simulink model "test_mdl_NI"  (R2018a)
settings: Solver=VariableStepAuto  StartTime=0.0  StopTime=10.0  RelTol=1e-3
(part 16 of 24)

== system test_mdl_NI/CAN_Signal/ABS_ESC/TrailerBrakeData_0x412/VehPtch_An_Dsply ==
  in : Inport
  out : Outport
  wires:
  in/1 -> out/1

== system test_mdl_NI/CAN_Signal/ABS_ESC/TrailerBrakeData_0x412/VehRol_An_Dsply ==
  in : Inport
  out : Outport
  wires:
  in/1 -> out/1

== system test_mdl_NI/CAN_Signal/ABS_ESC/WheelData_0x216/BrkObdData_No_Actl ==
  in : Inport
  out : Outport
  wires:
  in/1 -> out/1

== system test_mdl_NI/CAN_Signal/ABS_ESC/WheelData_0x216/BrkObdIndex_No_Actl ==
  in : Inport
  out : Outport
  wires:
  in/1 -> out/1

== system test_mdl_NI/CAN_Signal/ABS_ESC/WheelData_0x216/WhlDirFl_D_Actl ==
  in : Inport
  out : Outport
  wires:
  in/1 -> out/1

== system test_mdl_NI/CAN_Signal/ABS_ESC/WheelData_0x216/WhlDirFr_D_Actl ==
  in : Inport
  out : Outport
  wires:
  in/1 -> out/1

== system test_mdl_NI/CAN_Signal/ABS_ESC/WheelData_0x216/WhlDirRl_D_Actl ==
  in : Inport
  out : Outport
  wires:
  in/1 -> out/1

== system test_mdl_NI/CAN_Signal/ABS_ESC/WheelData_0x216/WhlDirRr_D_Actl ==
  in : Inport
  out : Outport
  wires:
  in/1 -> out/1

== system test_mdl_NI/CAN_Signal/ABS_ESC/WheelData_0x216/WhlRotatFl_No_Cnt ==
  in : Inport
  out : Outport
  wires:
  in/1 -> out/1

== system test_mdl_NI/CAN_Signal/ABS_ESC/WheelData_0x216/WhlRotatFr_No_Cnt ==
  in : Inport
  out : Outport
  wires:
  in/1 -> out/1

== system test_mdl_NI/CAN_Signal/ABS_ESC/WheelData_0x216/WhlRotatRl_No_Cnt ==
  in : Inport
  out : Outport
  wires:
  in/1 -> out/1

== system test_mdl_NI/CAN_Signal/ABS_ESC/WheelData_0x216/WhlRotatRr_No_Cnt ==
  in : Inport
  out : Outport
  wires:
  in/1 -> out/1

== system test_mdl_NI/CAN_Signal/ABS_ESC/WheelSpeed_0x217/WhlFl_W_Meas ==
  in : Inport
  out : Outport
  wires:
  in/1 -> out/1

== system test_mdl_NI/CAN_Signal/ABS_ESC/WheelSpeed_0x217/WhlFr_W_Meas ==
  in : Inport
  out : Outport
  wires:
  in/1 -> out/1

== system test_mdl_NI/CAN_Signal/ABS_ESC/WheelSpeed_0x217/WhlRl_W_Meas ==
  in : Inport
  out : Outport
  wires:
  in/1 -> out/1

== system test_mdl_NI/CAN_Signal/ABS_ESC/WheelSpeed_0x217/WhlRr_W_Meas ==
  in : Inport
  out : Outport
  wires:
  in/1 -> out/1

== system test_mdl_NI/CAN_Signal/ADAS/ACCDATA/AccBrkDecel_B_Rq ==
  in : Inport
  out : Outport
  wires:
  in/1 -> out/1

== system test_mdl_NI/CAN_Signal/ADAS/ACCDATA/AccBrkPrchg_B_Rq ==
  in : Inport
  out : Outport
  wires:
  in/1 -> out/1

== system test_mdl_NI/CAN_Signal/ADAS/ACCDATA/AccBrkTot_A_Rq ==
  in : Inport
  out : Outport
  wires:
  in/1 -> out/1

== system test_mdl_NI/CAN_Signal/ADAS/ACCDATA/AccCancl_B_Rq ==
  in : Inport
  out : Outport
  wires:
  in/1 -> out/1

== system test_mdl_NI/CAN_Signal/ADAS/ACCDATA/AccPrpl_A_Rq ==
  in : Inport
  out : Outport
  wires:
  in/1 -> out/1

== system test_mdl_NI/CAN_Signal/ADAS/ACCDATA/AccPrpl_A_Rq1 ==
  in : Inport
  out : Outport
  wires:
  in/1 -> out/1

== system test_mdl_NI/CAN_Signal/ADAS/ACCDATA/AccStopStat_B_Rq ==
  in : Inport
  out : Outport
  wires:
  in/1 -> out/1

== system test_mdl_NI/CAN_Signal/ADAS/ACCDATA/CmbbEngTqMn_B_Rq ==
  in : Inport
  out : Outport
  wires:
  in/1 -> out/1

== system test_mdl_NI/CAN_Signal/ADAS/ACCDATA_2/CmbbBaSens_D_Rq ==
  in : Inport
  out : Outport
  wires:
  in/1 -> out/1

== system test_mdl_NI/CAN_Signal/ADAS/ACCDATA_2/CmbbBrkDecel_A_Rq ==
  in : Inport
  out : Outport
  wires:
  in/1 -> out/1

== system test_mdl_NI/CAN_Signal/ADAS/ACCDATA_2/CmbbBrkDecel_B_Rq ==
  in : Inport
  out : Outport
  wires:
  in/1 -> out/1

== system test_mdl_NI/CAN_Signal/ADAS/ACCDATA_2/CmbbBrkPrchg_D_Rq ==
  in : Inport
  out : Outport
  wires:
  in/1 -> out/1

== system test_mdl_NI/CAN_Signal/BCM/BCM_Lamp_Stat_0x3C3/BrkWarnInd_B_Rq ==
  in : Inport
  out : Outport
  wires:
  in/1 -> out/1

== system test_mdl_NI/CAN_Signal/BCM/BCM_Lamp_Stat_0x3C3/Brk_Fluid_Lvl_Low ==
  in : Inport
  out : Outport
  wires:
  in/1 -> out/1

== system test_mdl_NI/CAN_Signal/BCM/BCM_Lamp_Stat_0x3C3/Courtesy_BSave_Stat ==
  in : Inport
  out : Outport
  wires:
  in/1 -> out/1

== system test_mdl_NI/CAN_Signal/BCM/BCM_Lamp_Stat_0x3C3/Courtesy_Delay_Status ==
  in : Inport
  out : Outport
  wires:
  in/1 -> out/1

== system test_mdl_NI/CAN_Signal/BCM/BCM_Lamp_Stat_0x3C3/CrnrLghtLeft_Pc_Rq ==
  in : Inport
  out : Outport
  wires:
  in/1 -> out/1

== system test_mdl_NI/CAN_Signal/BCM/BCM_Lamp_Stat_0x3C3/CrnrLghtRight_Pc_Rq ==
  in : Inport
  out : Outport
  wires:
  in/1 -> out/1

== system test_mdl_NI/CAN_Signal/BCM/BCM_Lamp_Stat_0x3C3/DayRnngLampOn_B_Stat ==
  in : Inport
  out : Outport
  wires:
  in/1 -> out/1

== system test_mdl_NI/CAN_Signal/BCM/BCM_Lamp_Stat_0x3C3/DrTgateLck_D_Stat ==
  in : Inport
  out : Outport
  wires:
  in/1 -> out/1

== system test_mdl_NI/CAN_Signal/BCM/BCM_Lamp_Stat_0x3C3/Dr_Courtesy_Light_Stat ==
  in : Inport
  out : Outport
  wires:
  in/1 -> out/1

== system test_mdl_NI/CAN_Signal/BCM/BCM_Lamp_Stat_0x3C3/HeadLampLoActv_B_Stat ==
  in : Inport
  out : Outport
  wires:
  in/1 -> out/1

== system test_mdl_NI/CAN_Signal/BCM/BCM_Lamp_Stat_0x3C3/HeadLampLoFlOn_B_Stat ==
  in : Inport
  out : Outport
  wires:
  in/1 -> out/1

== system test_mdl_NI/CAN_Signal/BCM/BCM_Lamp_Stat_0x3C3/HeadLampLoFrOn_B_Stat ==
  in : Inport
  out : Outport
  wires:
  in/1 -> out/1

== system test_mdl_NI/CAN_Signal/BCM/BCM_Lamp_Stat_0x3C3/HeadLampLoOut_B_Stat ==
  in : Inport
  out : Outport
  wires:
  in/1 -> out/1

== system test_mdl_NI/CAN_Signal/BCM/BCM_Lamp_Stat_0x3C3/HeadLghtHiFdbck_D_Stat ==
  in : Inport
  out : Outport
  wires:
  in/1 -> out/1

== system test_mdl_NI/CAN_Signal/BCM/BCM_Lamp_Stat_0x3C3/HeadLghtHiOn_B_Stat ==
  in : Inport
  out : Outport
  wires:
  in/1 -> out/1

== system test_mdl_NI/CAN_Signal/BCM/BCM_Lamp_Stat_0x3C3/HeadLghtSwtch_D_Stat ==
  in : Inport
  out : Outport
  wires:
  in/1 -> out/1

== system test_mdl_NI/CAN_Signal/BCM/BCM_Lamp_Stat_0x3C3/Headlamp_On_Wrning_Cmd ==
  in : Inport
  out : Outport
  wires:
  in/1 -> out/1

== system test_mdl_NI/CAN_Signal/BCM/BCM_Lamp_Stat_0x3C3/HomeSafeLtChime_B_Rq ==
  in : Inport
  out : Outport
  wires:
  in/1 -> out/1

== system test_mdl_NI/CAN_Signal/BCM/BCM_Lamp_Stat_0x3C3/Illuminated_Entry_Stat ==
  in : Inport
  out : Outport
  wires:
  in/1 -> out/1

== system test_mdl_NI/CAN_Signal/BCM/BCM_Lamp_Stat_0x3C3/ImpactEvntFdbck_D_Stat ==
  in : Inport
  out : Outport
  wires:
  in/1 -> out/1

== system test_mdl_NI/CAN_Signal/BCM/BCM_Lamp_Stat_0x3C3/KeyInIgnWarn_B_Cmd ==
  in : Inport
  out : Outport
  wires:
  in/1 -> out/1

== system test_mdl_NI/CAN_Signal/BCM/BCM_Lamp_Stat_0x3C3/Park_Brake_Chime_Rqst ==
  in : Inport
  out : Outport
  wires:
  in/1 -> out/1

== system test_mdl_NI/CAN_Signal/BCM/BCM_Lamp_Stat_0x3C3/PerimeterAlarmChimeRq ==
  in : Inport
  out : Outport
  wires:
  in/1 -> out/1

== system test_mdl_NI/CAN_Signal/BCM/BCM_Lamp_Stat_0x3C3/Perimeter_Alarm_Status ==
  in : Inport
  out : Outport
  wires:
  in/1 -> out/1

== system test_mdl_NI/CAN_Signal/BCM/BCM_Lamp_Stat_0x3C3/PrkLght_D_Stat ==
  in : Inport
  out : Outport
  wires:
  in/1 -> out/1

== system test_mdl_NI/CAN_Signal/BCM/BCM_Lamp_Stat_0x3C3/PrkLightChime_B_Rq ==
  in : Inport
  out : Outport
  wires:
  in/1 -> out/1

== system test_mdl_NI/CAN_Signal/BCM/BCM_Lamp_Stat_0x3C3/PudLampDrv_D_Rq ==
  in : Inport
  out : Outport
  wires:
  in/1 -> out/1

== system test_mdl_NI/CAN_Signal/BCM/BCM_Lamp_Stat_0x3C3/PudLampPsngr_D_Rq ==
  in : Inport
  out : Outport
  wires:
  in/1 -> out/1

== system test_mdl_NI/CAN_Signal/BCM/BCM_Lamp_Stat_0x3C3/PudLamp_D_Rq ==
  in : Inport
  out : Outport
  wires:
  in/1 -> out/1

== system test_mdl_NI/CAN_Signal/BCM/BCM_Lamp_Stat_0x3C3/ReducedGuard_D_Stat ==
  in : Inport
  out : Outport
  wires:
  in/1 -> out/1

== system test_mdl_NI/CAN_Signal/BCM/BCM_Lamp_Stat_0x3C3/RvrseLghtOn_B_Stat ==
  in : Inport
  out : Outport
  wires:
  in/1 -> out/1

== system test_mdl_NI/CAN_Signal/BCM/BCM_Lamp_Stat_0x3C3/StopLghtOn_B_Stat ==
  in : Inport
  out : Outport
  wires:
  in/1 -> out/1

== system test_mdl_NI/CAN_Signal/BCM/BCM_Lamp_Stat_0x3C3/TrnNotInPrkChime_B_Rq ==
  in : Inport
  out : Outport
  wires:
  in/1 -> out/1

== system test_mdl_NI/CAN_Signal/BCM/BCM_Lamp_Stat_0x3C3/WndwGlbl_D_Cmd ==
  in : Inport
  out : Outport
  wires:
  in/1 -> out/1

== system test_mdl_NI/CAN_Signal/BCM/BCM_Lamp_Stat_0x3C3/WrlssAcsyChrgInhbt_B_Rq ==
  in : Inport
  out : Outport
  wires:
  in/1 -> out/1

== system test_mdl_NI/CAN_Signal/BCM/Battery_Mgmt_24V_0x42E/BattULo24Soc_Pc_Actl ==
  in : Inport
  out : Outport
  wires:
  in/1 -> out/1

== system test_mdl_NI/CAN_Signal/BCM/Battery_Mgmt_24V_0x42E/BattULo24State_D_Qlty ==
  in : Inport
  out : Outport
  wires:
  in/1 -> out/1

== system test_mdl_NI/CAN_Signal/BCM/Battery_Mgmt_24V_0x42E/BattULo24_Ah_DeltaRide ==
  in : Inport
  out : Outport
  wires:
  in/1 -> out/1

== system test_mdl_NI/CAN_Signal/BCM/Battery_Mgmt_24V_0x42E/BattULo24_B_Falt ==
  in : Inport
  out : Outport
  wires:
  in/1 -> out/1

== system test_mdl_NI/CAN_Signal/BCM/Battery_Mgmt_24V_0x42E/BattULo24_I_Actl ==
  in : Inport
  out : Outport
  wires:
  in/1 -> out/1

== system test_mdl_NI/CAN_Signal/BCM/Battery_Mgmt_2_0x42C/BattULoChrg_D_Rq ==
  in : Inport
  out : Outport
  wires:
  in/1 -> out/1

== system test_mdl_NI/CAN_Signal/BCM/Battery_Mgmt_2_0x42C/BattULoSrvc_T_Actl ==
  in : Inport
  out : Outport
  wires:
  in/1 -> out/1

== system test_mdl_NI/CAN_Signal/BCM/Battery_Mgmt_2_0x42C/Batt_Crit_SoC_B ==
  in : Inport
  out : Outport
  wires:
  in/1 -> out/1

== system test_mdl_NI/CAN_Signal/BCM/Battery_Mgmt_2_0x42C/Batt_Lo_SoC_B ==
  in : Inport
  out : Outport
  wires:
  in/1 -> out/1

== system test_mdl_NI/CAN_Signal/BCM/Battery_Mgmt_2_0x42C/ChargeMode ==
  in : Inport
  out : Outport
  wires:
  in/1 -> out/1

== system test_mdl_NI/CAN_Signal/BCM/Battery_Mgmt_2_0x42C/EngStrtInhbt_B_RqBatt ==
  in : Inport
  out : Outport
  wires:
  in/1 -> out/1

== system test_mdl_NI/CAN_Signal/BCM/Battery_Mgmt_2_0x42C/IdleSpeedIncrease_El ==
  in : Inport
  out : Outport
  wires:
  in/1 -> out/1

== system test_mdl_NI/CAN_Signal/BCM/Battery_Mgmt_2_0x42C/PeriodicElLoad_B_Stat ==
  in : Inport
  out : Outport
  wires:
  in/1 -> out/1

== system test_mdl_NI/CAN_Signal/BCM/Battery_Mgmt_2_0x42C/PwSysULoFalt_D_Stat ==
  in : Inport
  out : Outport
  wires:
  in/1 -> out/1

== system test_mdl_NI/CAN_Signal/BCM/Battery_Mgmt_2_0x42C/Shed_Drain_Eng_Off_B ==
  in : Inport
  out : Outport
  wires:
  in/1 -> out/1

== system test_mdl_NI/CAN_Signal/BCM/Battery_Mgmt_2_0x42C/Shed_Feature_Group_ID ==
  in : Inport
  out : Outport
  wires:
  in/1 -> out/1

== system test_mdl_NI/CAN_Signal/BCM/Battery_Mgmt_2_0x42C/Shed_Level_Req ==
  in : Inport
  out : Outport
  wires:
  in/1 -> out/1

== system test_mdl_NI/CAN_Signal/BCM/Battery_Mgmt_2_0x42C/Shed_T_Eng_Off_B ==
  in : Inport
  out : Outport
  wires:
  in/1 -> out/1

== system test_mdl_NI/CAN_Signal/BCM/Battery_Mgmt_2_0x42C/ULoRgenTestMde_B_Rq ==
  in : Inport
  out : Outport
  wires:
  in/1 -> out/1

== system test_mdl_NI/CAN_Signal/BCM/Battery_Mgmt_3_0x43C/BSBattQCapAh ==
  in : Inport
  out : Outport
  wires:
  in/1 -> out/1

== system test_mdl_NI/CAN_Signal/BCM/Battery_Mgmt_3_0x43C/BSBattQDeltaRideAh ==
  in : Inport
  out : Outport
  wires:
  in/1 -> out/1

== system test_mdl_NI/CAN_Signal/BCM/Battery_Mgmt_3_0x43C/BSBattSOC ==
  in : Inport
  out : Outport
  wires:
  in/1 -> out/1

== system test_mdl_NI/CAN_Signal/BCM/Battery_Mgmt_3_0x43C/BSFault ==
  in : Inport
  out : Outport
  wires:
  in/1 -> out/1

== system test_mdl_NI/CAN_Signal/BCM/Battery_Mgmt_3_0x43C/BattULo2_Te_Actl ==
  in : Inport
  out : Outport
  wires:
  in/1 -> out/1

== system test_mdl_NI/CAN_Signal/BCM/Battery_Mgmt_3_0x43C/BattULoChrg_URate_RqMx ==
  in : Inport
  out : Outport
  wires:
  in/1 -> out/1

== system test_mdl_NI/CAN_Signal/BCM/Battery_Mgmt_3_0x43C/BattULoChrg_U_RqMn ==
  in : Inport
  out : Outport
  wires:
  in/1 -> out/1

== system test_mdl_NI/CAN_Signal/BCM/Battery_Mgmt_3_0x43C/BattULoChrg_U_RqMx ==
  in : Inport
  out : Outport
  wires:
  in/1 -> out/1

== system test_mdl_NI/CAN_Signal/BCM/Battery_Mgmt_3_0x43C/BattULoState_D_Qlty ==
  in : Inport
  out : Outport
  wires:
  in/1 -> out/1

== system test_mdl_NI/CAN_Signal/BCM/Battery_Mgmt_4_0x42B/BattULoAuxSoc_Pc_Actl ==
  in : Inport
  out : Outport
  wires:
  in/1 -> out/1

== system test_mdl_NI/CAN_Signal/BCM/Battery_Mgmt_4_0x42B/BattULoAux_B_Falt ==
  in : Inport
  out : Outport
  wires:
  in/1 -> out/1

== system test_mdl_NI/CAN_Signal/BCM/Battery_Mgmt_4_0x42B/BattULoAux_D_Qlty ==
  in : Inport
  out : Outport
  wires:
  in/1 -> out/1

== system test_mdl_NI/CAN_Signal/BCM/Battery_Mgmt_4_0x42B/BattULoAux_I_Actl ==
  in : Inport
  out : Outport
  wires:
  in/1 -> out/1

== system test_mdl_NI/CAN_Signal/BCM/Battery_Mgmt_4_0x42B/BattULoAux_U_Actl ==
  in : Inport
  out : Outport
  wires:
  in/1 -> out/1

== system test_mdl_NI/CAN_Signal/BCM/Battery_Mgmt_4_0x42B/BattULoCrnkBelt_U_Pred ==
  in : Inport
  out : Outport
  wires:
  in/1 -> out/1

== system test_mdl_NI/CAN_Signal/BCM/Battery_Mgmt_4_0x42B/BattULoCrnkStrt_U_Pred ==
  in : Inport
  out : Outport
  wires:
  in/1 -> out/1

== system test_mdl_NI/CAN_Signal/BCM/BodyInfo_3_0x3B3/Backlit_LED_Status ==
  in : Inport
  out : Outport
  wires:
  in/1 -> out/1

== system test_mdl_NI/CAN_Signal/BCM/BodyInfo_3_0x3B3/BodySrvcRqd_B_Rq ==
  in : Inport
  out : Outport
  wires:
  in/1 -> out/1

== system test_mdl_NI/CAN_Signal/BCM/BodyInfo_3_0x3B3/CrashEvnt_D_Stat ==
  in : Inport
  out : Outport
  wires:
  in/1 -> out/1

== system test_mdl_NI/CAN_Signal/BCM/BodyInfo_3_0x3B3/Day_Night_Status ==
  in : Inport
  out : Outport
  wires:
  in/1 -> out/1

== system test_mdl_NI/CAN_Signal/BCM/BodyInfo_3_0x3B3/Delay_Accy ==
  in : Inport
  out : Outport
  wires:
  in/1 -> out/1

== system test_mdl_NI/CAN_Signal/BCM/BodyInfo_3_0x3B3/DimmingLvlEvnt_No_Actl ==
  in : Inport
  out : Outport
  wires:
  in/1 -> out/1

== system test_mdl_NI/CAN_Signal/BCM/BodyInfo_3_0x3B3/Dimming_Lvl ==
  in : Inport
  out : Outport
  wires:
  in/1 -> out/1

== system test_mdl_NI/CAN_Signal/BCM/BodyInfo_3_0x3B3/DrStatDrvErrCnt_B_Stat ==
  in : Inport
  out : Outport
  wires:
  in/1 -> out/1

== system test_mdl_NI/CAN_Signal/BCM/BodyInfo_3_0x3B3/DrStatDrv_B_Actl ==
  in : Inport
  out : Outport
  wires:
  in/1 -> out/1

== system test_mdl_NI/CAN_Signal/BCM/BodyInfo_3_0x3B3/DrStatHood_B_Actl ==
  in : Inport
  out : Outport
  wires:
  in/1 -> out/1

== system test_mdl_NI/CAN_Signal/BCM/BodyInfo_3_0x3B3/DrStatInnrTgate_B_Actl ==
  in : Inport
  out : Outport
  wires:
  in/1 -> out/1

== system test_mdl_NI/CAN_Signal/BCM/BodyInfo_3_0x3B3/DrStatPsngr_B_Actl ==
  in : Inport
  out : Outport
  wires:
  in/1 -> out/1

== system test_mdl_NI/CAN_Signal/BCM/BodyInfo_3_0x3B3/DrStatRl_B_Actl ==
  in : Inport
  out : Outport
  wires:
  in/1 -> out/1

== system test_mdl_NI/CAN_Signal/BCM/BodyInfo_3_0x3B3/DrStatRr_B_Actl ==
  in : Inport
  out : Outport
  wires:
  in/1 -> out/1

== system test_mdl_NI/CAN_Signal/BCM/BodyInfo_3_0x3B3/DrStatTgate_B_Actl ==
  in : Inport
  out : Outport
  wires:
  in/1 -> out/1

== system test_mdl_NI/CAN_Signal/BCM/BodyInfo_3_0x3B3/FogLghtFrontOn_B_Stat ==
  in : Inport
  out : Outport
  wires:
  in/1 -> out/1

== system test_mdl_NI/CAN_Signal/BCM/BodyInfo_3_0x3B3/FogLghtRearOn_B_Stat ==
  in : Inport
  out : Outport
  wires:
  in/1 -> out/1

== system test_mdl_NI/CAN_Signal/BCM/BodyInfo_3_0x3B3/FuelPmpInhbt_B_Stat ==
  in : Inport
  out : Outport
  wires:
  in/1 -> out/1

== system test_mdl_NI/CAN_Signal/BCM/BodyInfo_3_0x3B3/IgnKeyType_D_Actl ==
  in : Inport
  out : Outport
  wires:
  in/1 -> out/1

== system test_mdl_NI/CAN_Signal/BCM/BodyInfo_3_0x3B3/Ignition_Status ==
  in : Inport
  out : Outport
  wires:
  in/1 -> out/1

== system test_mdl_NI/CAN_Signal/BCM/BodyInfo_3_0x3B3/Key_In_Ignition_Stat ==
  in : Inport
  out : Outport
  wires:
  in/1 -> out/1

== system test_mdl_NI/CAN_Signal/BCM/BodyInfo_3_0x3B3/LifeCycMde_D_Actl ==
  in : Inport
  out : Outport
  wires:
  in/1 -> out/1

== system test_mdl_NI/CAN_Signal/BCM/BodyInfo_3_0x3B3/Litval ==
  in : Inport
  out : Outport
  wires:
  in/1 -> out/1

== system test_mdl_NI/CAN_Signal/BCM/BodyInfo_3_0x3B3/Parklamp_Status ==
  in : Inport
  out : Outport
  wires:
  in/1 -> out/1

== system test_mdl_NI/CAN_Signal/BCM/BodyInfo_3_0x3B3/PrkBrkActv_B_Actl ==
  in : Inport
  out : Outport
  wires:
  in/1 -> out/1

== system test_mdl_NI/CAN_Signal/BCM/BodyInfo_3_0x3B3/Remote_Start_Status ==
  in : Inport
  out : Outport
  wires:
  in/1 -> out/1

== system test_mdl_NI/CAN_Signal/BCM/BodyInfo_3_0x3B3/TurnLghtLeftOn_B_Stat ==
  in : Inport
  out : Outport
  wires:
  in/1 -> out/1

== system test_mdl_NI/CAN_Signal/BCM/BodyInfo_3_0x3B3/TurnLghtLeft_D_Rq ==
  in : Inport
  out : Outport
  wires:
  in/1 -> out/1

== system test_mdl_NI/CAN_Signal/BCM/BodyInfo_3_0x3B3/TurnLghtRightOn_B_Stat ==
  in : Inport
  out : Outport
  wires:
  in/1 -> out/1

== system test_mdl_NI/CAN_Signal/BCM/BodyInfo_3_0x3B3/TurnLghtRight_D_Rq ==
  in : Inport
  out : Outport
  wires:
  in/1 -> out/1

== system test_mdl_NI/CAN_Signal/BCM/BodyInfo_3_0x3B3/ValetMode_D_Mem ==
  in : Inport
  out : Outport
  wires:
  in/1 -> out/1

== system test_mdl_NI/CAN_Signal/BCM/Body_Info_10_0x3BA/GenericSwtch1_No_Actl ==
  in : Inport
  out : Outport
  wires:
  in/1 -> out/1

== system test_mdl_NI/CAN_Signal/BCM/Body_Info_10_0x3BA/GenericSwtch2_No_Actl ==
  in : Inport
  out : Outport
  wires:
  in/1 -> out/1

== system test_mdl_NI/CAN_Signal/BCM/Body_Info_10_0x3BA/GenericSwtch3_No_Actl ==
  in : Inport
  out : Outport
  wires:
  in/1 -> out/1

== system test_mdl_NI/CAN_Signal/BCM/Body_Info_12_0x26E/FobCtlPssvData_No_Actl ==
  in : Inport
  out : Outport
  wires:
  in/1 -> out/1

== system test_mdl_NI/CAN_Signal/BCM/Body_Info_12_0x26E/FobCtlRollCode_No_Stat ==
  in : Inport
  out : Outport
  wires:
  in/1 -> out/1

== system test_mdl_NI/CAN_Signal/BCM/Body_Info_12_0x26E/FobCtlType_D_Stat ==
  in : Inport
  out : Outport
  wires:
  in/1 -> out/1

== system test_mdl_NI/CAN_Signal/BCM/Body_Info_4_0x242/BattULo_I_Actl ==
  in : Inport
  out : Outport
  wires:
  in/1 -> out/1

== system test_mdl_NI/CAN_Signal/BCM/Body_Info_4_0x242/BattULo_U_Actl ==
  in : Inport
  out : Outport
  wires:
  in/1 -> out/1

== system test_mdl_NI/CAN_Signal/BCM/Body_Info_4_0x242/BrkTrnShifLck_B_Stat ==
  in : Inport
  out : Outport
  wires:
  in/1 -> out/1

== system test_mdl_NI/CAN_Signal/BCM/Body_Info_4_0x242/DcacElPw_D_Rq ==
  in : Inport
  out : Outport
  wires:
  in/1 -> out/1

== system test_mdl_NI/CAN_Signal/BCM/Body_Info_4_0x242/DriverCrankingReq ==
  in : Inport
  out : Outport
  wires:
  in/1 -> out/1

== system test_mdl_NI/CAN_Signal/BCM/Body_Info_4_0x242/EngOff_T_Actl ==
  in : Inport
  out : Outport
  wires:
  in/1 -> out/1

== system test_mdl_NI/CAN_Signal/BCM/Body_Info_4_0x242/FuelPumpPwr_D_Stat ==
  in : Inport
  out : Outport
  wires:
  in/1 -> out/1

== system test_mdl_NI/CAN_Signal/BCM/Body_Info_4_0x242/PrkLckCtlAvail_T_Stat ==
  in : Inport
  out : Outport
  wires:
  in/1 -> out/1

== system test_mdl_NI/CAN_Signal/BCM/Body_Info_4_0x242/PrkLckCtlMsgTxt_D_Rq ==
  in : Inport
  out : Outport
  wires:
  in/1 -> out/1

== system test_mdl_NI/CAN_Signal/BCM/Body_Info_4_0x242/PrkLckCtlTow_B_Enbl ==
  in : Inport
  out : Outport
  wires:
  in/1 -> out/1

== system test_mdl_NI/CAN_Signal/BCM/Body_Info_4_0x242/PrkLckCtlUnlck_D_Stat ==
  in : Inport
  out : Outport
  wires:
  in/1 -> out/1

== system test_mdl_NI/CAN_Signal/BCM/Body_Info_4_0x242/PrkLckCtl_B_Enbl ==
  in : Inport
  out : Outport
  wires:
  in/1 -> out/1

== system test_mdl_NI/CAN_Signal/BCM/Body_Info_4_0x242/PtLatchActv_B_RqBcm ==
  in : Inport
  out : Outport
  wires:
  in/1 -> out/1

== system test_mdl_NI/CAN_Signal/BCM/Body_Info_4_0x242/ReFuelSwtchStat_D_Actl ==
  in : Inport
  out : Outport
  wires:
  in/1 -> out/1

== system test_mdl_NI/CAN_Signal/BCM/Body_Info_4_0x242/immoSecureIdleMode ==
  in : Inport
  out : Outport
  wires:
  in/1 -> out/1

== system test_mdl_NI/CAN_Signal/BCM/Body_Info_6_0x38D/DrLatchMsgTxt_D_Rq ==
  in : Inport
  out : Outport
  wires:
  in/1 -> out/1

== system test_mdl_NI/CAN_Signal/BCM/Body_Info_6_0x38D/ElPwPoint_D_Rq ==
  in : Inport
  out : Outport
  wires:
  in/1 -> out/1

== system test_mdl_NI/CAN_Signal/BCM/Body_Info_6_0x38D/HeadLghtHiPrmsn_D_Stat ==
  in : Inport
  out : Outport
  wires:
  in/1 -> out/1

== system test_mdl_NI/CAN_Signal/BCM/Body_Info_6_0x38D/IgnPsswrdDsply_B_Rq ==
  in : Inport
  out : Outport
  wires:
  in/1 -> out/1

== system test_mdl_NI/CAN_Signal/BCM/Body_Info_6_0x38D/KeyAdmnTot_No_Cnt ==
  in : Inport
  out : Outport
  wires:
  in/1 -> out/1

== system test_mdl_NI/CAN_Signal/BCM/Body_Info_6_0x38D/KeyMykeyTot_No_Cnt ==
  in : Inport
  out : Outport
  wires:
  in/1 -> out/1

== system test_mdl_NI/CAN_Signal/BCM/Body_Info_6_0x38D/Keycode_Status ==
  in : Inport
  out : Outport
  wires:
  in/1 -> out/1

== system test_mdl_NI/CAN_Signal/BCM/Body_Info_6_0x38D/PEBackupSlot_Stats ==
  in : Inport
  out : Outport
  wires:
  in/1 -> out/1

== system test_mdl_NI/CAN_Signal/BCM/Body_Info_6_0x38D/PoliceIdlMde_D_Stat ==
  in : Inport
  out : Outport
  wires:
  in/1 -> out/1

== system test_mdl_NI/CAN_Signal/BCM/Body_Info_6_0x38D/PrmtrAlrmEvnt_D_Stat ==
  in : Inport
  out : Outport
  wires:
  in/1 -> out/1

== system test_mdl_NI/CAN_Signal/BCM/Body_Info_6_0x38D/PrsnlDevcChrgEnbl_B_Rq ==
  in : Inport
  out : Outport
  wires:
  in/1 -> out/1

== system test_mdl_NI/CAN_Signal/BCM/Body_Info_6_0x38D/SecurityMsgTxt_D_Rq ==
  in : Inport
  out : Outport
  wires:
  in/1 -> out/1

== system test_mdl_NI/CAN_Signal/BCM/Body_Info_6_0x38D/SteWhlLckMsgTxt_D_Rq ==
  in : Inport
  out : Outport
  wires:
  in/1 -> out/1

== system test_mdl_NI/CAN_Signal/BCM/Body_Info_6_0x38D/TracKeyMde_D_Stat ==
  in : Inport
  out : Outport
  wires:
  in/1 -> out/1

== system test_mdl_NI/CAN_Signal/BCM/Body_Info_6_0x38D/immoMsgTxt_D_Rq ==
  in : Inport
  out : Outport
  wires:
  in/1 -> out/1

== system test_mdl_NI/CAN_Signal/BCM/Body_Info_7_0x3B1/KeyOffMde_D_Actl ==
  in : Inport
  out : Outport
  wires:
  in/1 -> out/1

== system test_mdl_NI/CAN_Signal/BCM/Body_Info_8_0x3B9/ChrgCordLck_B_Stat ==
  in : Inport
  out : Outport
  wires:
  in/1 -> out/1

== system test_mdl_NI/CAN_Signal/BCM/Body_Info_8_0x3B9/ChrgCordResp1_No_Actl ==
  in : Inport
  out : Outport
  wires:
  in/1 -> out/1

== system test_mdl_NI/CAN_Signal/BCM/Body_Info_8_0x3B9/ChrgCordResp2_No_Actl ==
  in : Inport
  out : Outport
  wires:
  in/1 -> out/1

== system test_mdl_NI/CAN_Signal/BCM/Body_Info_8_0x3B9/WakeAlarm0_D_Stat ==
  in : Inport
  out : Outport
  wires:
  in/1 -> out/1

== system test_mdl_NI/CAN_Signal/BCM/Body_Info_8_0x3B9/WakeAlarm1_D_Stat ==
  in : Inport
  out : Outport
  wires:
  in/1 -> out/1

== system test_mdl_NI/CAN_Signal/BCM/Body_Info_8_0x3B9/WakeAlarm2_D_Stat ==
  in : Inport
  out : Outport
  wires:
  in/1 -> out/1

== system test_mdl_NI/CAN_Signal/BCM/Body_Info_8_0x3B9/WakeAlarm3_D_Stat ==
  in : Inport
  out : Outport
  wires:
  in/1 -> out/1

== system test_mdl_NI/CAN_Signal/BCM/Body_Info_9_0x3A3/AdvStrt_D_Stat ==
  in : Inport
  out : Outport
  wires:
  in/1 -> out/1

== system test_mdl_NI/CAN_Signal/BCM/Body_Info_9_0x3A3/CrnkInhbt_B_Stat ==
  in : Inport
  out : Outport
  wires:
  in/1 -> out/1

== system test_mdl_NI/CAN_Signal/BCM/Body_Info_9_0x3A3/CrnkInhbt_No_Cnt ==
  in : Inport
  out : Outport
  wires:
  in/1 -> out/1

== system test_mdl_NI/CAN_Signal/BCM/Body_Info_9_0x3A3/CrnkInhbt_No_Cs ==
  in : Inport
  out : Outport
  wires:
  in/1 -> out/1

== system test_mdl_NI/CAN_Signal/BCM/Body_Info_9_0x3A3/DrvInCtl_B_Stat ==
  in : Inport
  out : Outport
  wires:
  in/1 -> out/1

== system test_mdl_NI/CAN_Signal/BCM/Body_Info_9_0x3A3/EngStrtActv_B_Stat ==
  in : Inport
  out : Outport
  wires:
  in/1 -> out/1

== system test_mdl_NI/CAN_Signal/BCM/Body_Info_9_0x3A3/EngStrt_B_Rq ==
  in : Inport
  out : Outport
  wires:
  in/1 -> out/1

== system test_mdl_NI/CAN_Signal/BCM/Body_Info_9_0x3A3/IgnPreOffActv_B_Stat ==
  in : Inport
  out : Outport
  wires:
  in/1 -> out/1

== system test_mdl_NI/CAN_Signal/BCM/Body_Info_9_0x3A3/StrtrMtrCtlDStat_No_Cs ==
  in : Inport
  out : Outport
  wires:
  in/1 -> out/1

== system test_mdl_NI/CAN_Signal/BCM/Body_Info_9_0x3A3/VehOnSrc_D_Stat ==
  in : Inport
  out : Outport
  wires:
  in/1 -> out/1

== system test_mdl_NI/CAN_Signal/BCM/CMPS_FDM_Info_Status_0x3C7/CamPDCGuidStat ==
  in : Inport
  out : Outport
  wires:
  in/1 -> out/1

== system test_mdl_NI/CAN_Signal/BCM/CMPS_FDM_Info_Status_0x3C7/CamZoomActiveState ==
  in : Inport
  out : Outport
  wires:
  in/1 -> out/1

== system test_mdl_NI/CAN_Signal/BCM/CMPS_FDM_Info_Status_0x3C7/CamraOvrlDyn_D_Actl ==
  in : Inport
  out : Outport
  wires:
  in/1 -> out/1

== system test_mdl_NI/CAN_Signal/BCM/CMPS_FDM_Info_Status_0x3C7/CamraOvrlStat_D_Actl ==
  in : Inport
  out : Outport
  wires:
  in/1 -> out/1

== system test_mdl_NI/CAN_Signal/BCM/CMPS_FDM_Info_Status_0x3C7/CamraOvrlTow_D_Actl ==
  in : Inport
  out : Outport
  wires:
  in/1 -> out/1

== system test_mdl_NI/CAN_Signal/BCM/CMPS_FDM_Info_Status_0x3C7/CamraViewSplit_D_Actl ==
  in : Inport
  out : Outport
  wires:
  in/1 -> out/1

== system test_mdl_NI/CAN_Signal/BCM/CMPS_FDM_Info_Status_0x3C7/CamraZoomMan_D_Actl ==
  in : Inport
  out : Outport
  wires:
  in/1 -> out/1

== system test_mdl_NI/CAN_Signal/BCM/CellPhonePassport_Stat_1_0x447/HeadLghtOn_D_Rq ==
  in : Inport
  out : Outport
  wires:
  in/1 -> out/1

== system test_mdl_NI/CAN_Signal/BCM/CellPhonePassport_Stat_1_0x447/KeyProg_No_Actl ==
  in : Inport
  out : Outport
  wires:
  in/1 -> out/1

== system test_mdl_NI/CAN_Signal/BCM/CellPhonePassport_Stat_1_0x447/PepsKeyActv_D_Stat ==
  in : Inport
  out : Outport
  wires:
  in/1 -> out/1

== system test_mdl_NI/CAN_Signal/BCM/CellPhonePassport_Stat_1_0x447/PepsKeyFound_No_Actl ==
  in : Inport
  out : Outport
  wires:
  in/1 -> out/1

== system test_mdl_NI/CAN_Signal/BCM/CellPhonePassport_Stat_1_0x447/Pers1Phone_D_Stat ==
  in : Inport
  out : Outport
  wires:
  in/1 -> out/1

== system test_mdl_NI/CAN_Signal/BCM/CellPhonePassport_Stat_1_0x447/Pers2Phone_D_Stat ==
  in : Inport
  out : Outport
  wires:
  in/1 -> out/1

== system test_mdl_NI/CAN_Signal/BCM/CellPhonePassport_Stat_1_0x447/Pers3Phone_D_Stat ==
  in : Inport
  out : Outport
  wires:
  in/1 -> out/1

== system test_mdl_NI/CAN_Signal/BCM/CellPhonePassport_Stat_1_0x447/Pers4Phone_D_Stat ==
  in : Inport
  out : Outport
  wires:
  in/1 -> out/1

== system test_mdl_NI/CAN_Signal/BCM/CellPhonePassport_Stat_1_0x447/RstrtSetting_T_Actl ==
  in : Inport
  out : Outport
  wires:
  in/1 -> out/1

== system test_mdl_NI/CAN_Signal/BCM/CellPhonePassport_Stat_1_0x447/Rstrt_T_Actl ==
  in : Inport
  out : Outport
  wires:
  in/1 -> out/1

== system test_mdl_NI/CAN_Signal/BCM/CellPhonePassport_Stat_1_0x447/VehLck_D_Dsply ==
  in : Inport
  out : Outport
  wires:
  in/1 -> out/1

== system test_mdl_NI/CAN_Signal/BCM/GGCC_Config_Mgmt_ID_1_0x40A/VehicleGGCCData ==
  in : Inport
  out : Outport
  wires:
  in/1 -> out/1

== system test_mdl_NI/CAN_Signal/BCM/GlobalClock_Data_0x84/GlblClkDay_No_Actl ==
  in : Inport
  out : Outport
  wires:
  in/1 -> out/1

== system test_mdl_NI/CAN_Signal/BCM/GlobalClock_Data_0x84/GlblClkHr_No_Actl ==
  in : Inport
  out : Outport
  wires:
  in/1 -> out/1

== system test_mdl_NI/CAN_Signal/BCM/GlobalClock_Data_0x84/GlblClkMnte_No_Actl ==
  in : Inport
  out : Outport
  wires:
  in/1 -> out/1

== system test_mdl_NI/CAN_Signal/BCM/GlobalClock_Data_0x84/GlblClkScnd_No_Actl ==
  in : Inport
  out : Outport
  wires:
  in/1 -> out/1

== system test_mdl_NI/CAN_Signal/BCM/GlobalClock_Data_0x84/GlblClkYr_No_Actl ==
  in : Inport
  out : Outport
  wires:
  in/1 -> out/1

== system test_mdl_NI/CAN_Signal/BCM/Global_PATS_Control_Info2_0x42/immoControlCmd_T2 ==
  in : Inport
  out : Outport
  wires:
  in/1 -> out/1

== system test_mdl_NI/CAN_Signal/BCM/Global_PATS_Control_Info2_0x42/immoControlData_T2 ==
  in : Inport
  out : Outport
  wires:
  in/1 -> out/1

== system test_mdl_NI/CAN_Signal/BCM/Global_PATS_Control_Info_0x41/immoControlCmd_T1 ==
  in : Inport
  out : Outport
  wires:
  in/1 -> out/1

== system test_mdl_NI/CAN_Signal/BCM/Global_PATS_Control_Info_0x41/immoControlData_T1 ==
  in : Inport
  out : Outport
  wires:
  in/1 -> out/1

== system test_mdl_NI/CAN_Signal/BCM/Locking_Systems_2_0x331/ChildLckMde_B_Stat ==
  in : Inport
  out : Outport
  wires:
  in/1 -> out/1

== system test_mdl_NI/CAN_Signal/BCM/Locking_Systems_2_0x331/ChildLck_D_Dsply ==
  in : Inport
  out : Outport
  wires:
  in/1 -> out/1

== system test_mdl_NI/CAN_Signal/BCM/Locking_Systems_2_0x331/DrTgateExtSwMde_B_Stat ==
  in : Inport
  out : Outport
  wires:
  in/1 -> out/1

== system test_mdl_NI/CAN_Signal/BCM/Locking_Systems_2_0x331/DrTgateOpen_B_Rq ==
  in : Inport
  out : Outport
  wires:
  in/1 -> out/1

== system test_mdl_NI/CAN_Signal/BCM/Locking_Systems_2_0x331/FobComm_D_Stat ==
  in : Inport
  out : Outport
  wires:
  in/1 -> out/1

== system test_mdl_NI/CAN_Signal/BCM/Locking_Systems_2_0x331/Keyfob_Pad_Msg_Count ==
  in : Inport
  out : Outport
  wires:
  in/1 -> out/1

== system test_mdl_NI/CAN_Signal/BCM/Locking_Systems_2_0x331/L_Pwr_Sliding_Dr_Rqst ==
  in : Inport
  out : Outport
  wires:
  in/1 -> out/1

== system test_mdl_NI/CAN_Signal/BCM/Locking_Systems_2_0x331/LockInhibit ==
  in : Inport
  out : Outport
  wires:
  in/1 -> out/1

== system test_mdl_NI/CAN_Signal/BCM/Locking_Systems_2_0x331/Lockmsgtxt_D_Rq ==
  in : Inport
  out : Outport
  wires:
  in/1 -> out/1

== system test_mdl_NI/CAN_Signal/BCM/Locking_Systems_2_0x331/Power_Decklid_Rqst ==
  in : Inport
  out : Outport
  wires:
  in/1 -> out/1

== system test_mdl_NI/CAN_Signal/BCM/Locking_Systems_2_0x331/Power_Liftgate_Rqst ==
  in : Inport
  out : Outport
  wires:
  in/1 -> out/1

== system test_mdl_NI/CAN_Signal/BCM/Locking_Systems_2_0x331/R_Pwr_Sliding_Dr_Rqst ==
  in : Inport
  out : Outport
  wires:
  in/1 -> out/1

== system test_mdl_NI/CAN_Signal/BCM/Locking_Systems_2_0x331/Remote_Device_Feedback ==
  in : Inport
  out : Outport
  wires:
  in/1 -> out/1

== system test_mdl_NI/CAN_Signal/BCM/Locking_Systems_2_0x331/RollCodeUnlock ==
  in : Inport
  out : Outport
  wires:
  in/1 -> out/1

== system test_mdl_NI/CAN_Signal/BCM/Locking_Systems_2_0x331/VehLckInd_D_Rq ==
  in : Inport
  out : Outport
  wires:
  in/1 -> out/1

== system test_mdl_NI/CAN_Signal/BCM/Locking_Systems_2_0x331/Veh_Lock_EvNum ==
  in : Inport
  out : Outport
  wires:
  in/1 -> out/1

== system test_mdl_NI/CAN_Signal/BCM/Locking_Systems_2_0x331/Veh_Lock_Requestor ==
  in : Inport
  out : Outport
  wires:
  in/1 -> out/1

== system test_mdl_NI/CAN_Signal/BCM/Locking_Systems_2_0x331/Veh_Lock_Status ==
  in : Inport
  out : Outport
  wires:
  in/1 -> out/1

== system test_mdl_NI/CAN_Signal/BCM/Locking_Systems_2_0x331/Veh_Lock_Sub_Id ==
  in : Inport
  out : Outport
  wires:
  in/1 -> out/1

== system test_mdl_NI/CAN_Signal/BCM/Locking_Systems_2_0x331/WindowLockout_B_Stat ==
  in : Inport
  out : Outport
  wires:
  in/1 -> out/1

== system test_mdl_NI/CAN_Signal/BCM/PaakRqData1_0x468/KeyPadCodeProg_D_Stat ==
  in : Inport
  out : Outport
  wires:
  in/1 -> out/1

== system test_mdl_NI/CAN_Signal/BCM/PaakRqData1_0x468/PaakTrgtData_D_Rq ==
  in : Inport
  out : Outport
  wires:
  in/1 -> out/1

== system test_mdl_NI/CAN_Signal/BCM/PaakRqData1_0x468/PaakTrgtPssvData_No_Rq ==
  in : Inport
  out : Outport
  wires:
  in/1 -> out/1

== system test_mdl_NI/CAN_Signal/BCM/PaakRqData1_0x468/PaakTrgtRollCode_No_Rq ==
  in : Inport
  out : Outport
  wires:
  in/1 -> out/1

== system test_mdl_NI/CAN_Signal/BCM/PaakRqData1_0x468/PaakTrgtType_D_Rq ==
  in : Inport
  out : Outport
  wires:
  in/1 -> out/1

== system test_mdl_NI/CAN_Signal/BCM/PaakRqData1_0x468/PaakTrgtZone_D_Rq ==
  in : Inport
  out : Outport
  wires:
  in/1 -> out/1

== system test_mdl_NI/CAN_Signal/BCM/PaakRqData2_0x469/PaakTrgtActvData_No_Rq ==
  in : Inport
  out : Outport
  wires:
  in/1 -> out/1

== system test_mdl_NI/CAN_Signal/BCM/Personality_BCM2_Data_0x3EB/AssocConfirm_D_Actl ==
  in : Inport
  out : Outport
  wires:
  in/1 -> out/1

== system test_mdl_NI/CAN_Signal/BCM/Personality_BCM2_Data_0x3EB/EmPrflKeyAssoc_D_Stat ==
  in : Inport
  out : Outport
  wires:
  in/1 -> out/1

== system test_mdl_NI/CAN_Signal/BCM/Personality_BCM2_Data_0x3EB/EmPrflNo_D_Stat ==
  in : Inport
  out : Outport
  wires:
  in/1 -> out/1

== system test_mdl_NI/CAN_Signal/BCM/Personality_BCM2_Data_0x3EB/Pers1Key_D_Stat ==
  in : Inport
  out : Outport
  wires:
  in/1 -> out/1

== system test_mdl_NI/CAN_Signal/BCM/Personality_BCM2_Data_0x3EB/Pers2Key_D_Stat ==
  in : Inport
  out : Outport
  wires:
  in/1 -> out/1

== system test_mdl_NI/CAN_Signal/BCM/Personality_BCM2_Data_0x3EB/Pers3Key_D_Stat ==
  in : Inport
  out : Outport
  wires:
  in/1 -> out/1

== system test_mdl_NI/CAN_Signal/BCM/Personality_BCM2_Data_0x3EB/Pers4Key_D_Stat ==
  in : Inport
  out : Outport
  wires:
  in/1 -> out/1

== system test_mdl_NI/CAN_Signal/BCM/Personality_BCM2_Data_0x3EB/PersConflict_D_Actl ==
  in : Inport
  out : Outport
  wires:
  in/1 -> out/1

== system test_mdl_NI/CAN_Signal/BCM/Personality_BCM2_Data_0x3EB/PersNoPos_D_Actl ==
  in : Inport
  out : Outport
  wires:
  in/1 -> out/1

== system test_mdl_NI/CAN_Signal/BCM/Personality_BCM2_Data_0x3EB/PersNo_D_Actl ==
  in : Inport
  out : Outport
  wires:
  in/1 -> out/1

== system test_mdl_NI/CAN_Signal/BCM/Personality_BCM2_Data_0x3EB/PersRecallSrc_D_Actl ==
  in : Inport
  out : Outport
  wires:
  in/1 -> out/1

== system test_mdl_NI/CAN_Signal/BCM/Personality_BCM2_Data_0x3EB/PersSetupAccessCtrl ==
  in : Inport
  out : Outport
  wires:
  in/1 -> out/1

== system test_mdl_NI/CAN_Signal/BCM/Personality_BCM2_Data_0x3EB/PersSetupRestr_D_Actl ==
  in : Inport
  out : Outport
  wires:
  in/1 -> out/1

== system test_mdl_NI/CAN_Signal/BCM/Personality_BCM2_Data_0x3EB/PersSetup_No_Actl ==
  in : Inport
  out : Outport
  wires:
  in/1 -> out/1

== system test_mdl_NI/CAN_Signal/BCM/Personality_BCM2_Data_0x3EB/RecallEvent_No_Cnt ==
  in : Inport
  out : Outport
  wires:
  in/1 -> out/1

== system test_mdl_NI/CAN_Signal/BCM/Personality_BCM2_Data_0x3EB/VehKeyActv_D_Stat ==
  in : Inport
  out : Outport
  wires:
  in/1 -> out/1

== system test_mdl_NI/CAN_Signal/BCM/Personality_BCM_Data_0x3E3/FeatConfigBcmActl ==
  in : Inport
  out : Outport
  wires:
  in/1 -> out/1

== system test_mdl_NI/CAN_Signal/BCM/Personality_BCM_Data_0x3E3/FeatNoBcm_No_Actl ==
  in : Inport
  out : Outport
  wires:
  in/1 -> out/1

== system test_mdl_NI/CAN_Signal/BCM/Personality_BCM_Data_0x3E3/FobAssocChime_B_Rq ==
  in : Inport
  out : Outport
  wires:
  in/1 -> out/1

== system test_mdl_NI/CAN_Signal/BCM/Personality_BCM_Data_0x3E3/LightAmbColor_No_Actl ==
  in : Inport
  out : Outport
  wires:
  in/1 -> out/1

== system test_mdl_NI/CAN_Signal/BCM/Personality_BCM_Data_0x3E3/LightAmbIntsty_No_Actl ==
  in : Inport
  out : Outport
  wires:
  in/1 -> out/1

== system test_mdl_NI/CAN_Signal/BCM/Personality_BCM_Data_0x3E3/PersIndexBcm_D_Actl ==
  in : Inport
  out : Outport
  wires:
  in/1 -> out/1

== system test_mdl_NI/CAN_Signal/BCM/Power_Stat_0x456/RstrnMdulePw_D_Falt ==
  in : Inport
  out : Outport
  wires:
  in/1 -> out/1

== system test_mdl_NI/CAN_Signal/BCM/RKE_Packet_0x3B6/Modulation_Ctrl ==
  in : Inport
  out : Outport
  wires:
  in/1 -> out/1

== system test_mdl_NI/CAN_Signal/BCM/RKE_Packet_0x3B6/RemoteKey_Info_Ctrl ==
  in : Inport
  out : Outport
  wires:
  in/1 -> out/1

== system test_mdl_NI/CAN_Signal/BCM/RKE_Packet_0x3B6/RemoteKey_Info_Index ==
  in : Inport
  out : Outport
  wires:
  in/1 -> out/1

== system test_mdl_NI/CAN_Signal/BCM/RKE_Packet_0x3B6/RemoteKey_Info_MaxInd ==
  in : Inport
  out : Outport
  wires:
  in/1 -> out/1

== system test_mdl_NI/CAN_Signal/BCM/RKE_Packet_0x3B6/RemoteKey_Info_TIC ==
  in : Inport
  out : Outport
  wires:
  in/1 -> out/1

== system test_mdl_NI/CAN_Signal/BCM/RKE_Packet_0x3B6/TirePress_Filter_Ctrl ==
  in : Inport
  out : Outport
  wires:
  in/1 -> out/1

== system test_mdl_NI/CAN_Signal/BCM/TPM_Frame_0x3B7/TirePress_Info_ID ==
  in : Inport
  out : Outport
  wires:
  in/1 -> out/1

== system test_mdl_NI/CAN_Signal/BCM/TPM_Frame_0x3B7/TirePress_Info_Index ==
  in : Inport
  out : Outport
  wires:
  in/1 -> out/1

== system test_mdl_NI/CAN_Signal/BCM/TPM_Frame_0x3B7/TirePress_Info_MaxInd ==
  in : Inport
  out : Outport
  wires:
  in/1 -> out/1

== system test_mdl_NI/CAN_Signal/BCM/Tire_Pressure_Data_0x3B5/Tire_Press_LF_Data ==
  in : Inport
  out : Outport
  wires:
  in/1 -> out/1

== system test_mdl_NI/CAN_Signal/BCM/Tire_Pressure_Data_0x3B5/Tire_Press_LR_OLR_Data ==
  in : Inport
  out : Outport
  wires:
  in/1 -> out/1

== system test_mdl_NI/CAN_Signal/BCM/Tire_Pressure_Data_0x3B5/Tire_Press_RF_Data ==
  in : Inport
  out : Outport
  wires:
  in/1 -> out/1

== system test_mdl_NI/CAN_Signal/BCM/Tire_Pressure_Data_0x3B5/Tire_Press_RR_ORR_Data ==
  in : Inport
  out : Outport
  wires:
  in/1 -> out/1

== system test_mdl_NI/CAN_Signal/BCM/Tire_Pressure_Data_DRW_0x3B8/Tire_Press_ILR_Data ==
  in : Inport
  out : Outport
  wires:
  in/1 -> out/1

== system test_mdl_NI/CAN_Signal/BCM/Tire_Pressure_Data_DRW_0x3B8/Tire_Press_IRR_Data ==
  in : Inport
  out : Outport
  wires:
  in/1 -> out/1

== system test_mdl_NI/CAN_Signal/BCM/Tire_Pressure_Stat_0x3B4/TirePReset_D_Stat ==
  in : Inport
  out : Outport
  wires:
  in/1 -> out/1

== system test_mdl_NI/CAN_Signal/BCM/Tire_Pressure_Stat_0x3B4/Tire_Press_ILR_Stat ==
  in : Inport
  out : Outport
  wires:
  in/1 -> out/1

== system test_mdl_NI/CAN_Signal/BCM/Tire_Pressure_Stat_0x3B4/Tire_Press_IRR_Stat ==
  in : Inport
  out : Outport
  wires:
  in/1 -> out/1

== system test_mdl_NI/CAN_Signal/BCM/Tire_Pressure_Stat_0x3B4/Tire_Press_LF_Stat ==
  in : Inport
  out : Outport
  wires:
  in/1 -> out/1

== system test_mdl_NI/CAN_Signal/BCM/Tire_Pressure_Stat_0x3B4/Tire_Press_LR_OLR_Stat ==
  in : Inport
  out : Outport
  wires:
  in/1 -> out/1

== system test_mdl_NI/CAN_Signal/BCM/Tire_Pressure_Stat_0x3B4/Tire_Press_Placrd_Frnt ==
  in : Inport
  out : Outport
  wires:
  in/1 -> out/1

== system test_mdl_NI/CAN_Signal/BCM/Tire_Pressure_Stat_0x3B4/Tire_Press_Placrd_Rear ==
  in : Inport
  out : Outport
  wires:
  in/1 -> out/1

== system test_mdl_NI/CAN_Signal/BCM/Tire_Pressure_Stat_0x3B4/Tire_Press_RF_Stat ==
  in : Inport
  out : Outport
  wires:
  in/1 -> out/1

== system test_mdl_NI/CAN_Signal/BCM/Tire_Pressure_Stat_0x3B4/Tire_Press_RR_ORR_Stat ==
  in : Inport
  out : Outport
  wires:
  in/1 -> out/1

== system test_mdl_NI/CAN_Signal/BCM/Tire_Pressure_Stat_0x3B4/Tire_Press_System_Stat ==
  in : Inport
  out : Outport
  wires:
  in/1 -> out/1

== system test_mdl_NI/CAN_Signal/BCM/Tire_Pressure_Stat_0x3B4/Tire_Press_Telltale ==
  in : Inport
  out : Outport
  wires:
  in/1 -> out/1

== system test_mdl_NI/CAN_Signal/DSMC/CMR_DSMC_AutoSar_NetwrkMgt/CMR_DSMC_AutoSarNMControl ==
  in : Inport
  out : Outport
  wires:
  in/1 -> out/1

== system test_mdl_NI/CAN_Signal/DSMC/CMR_DSMC_AutoSar_NetwrkMgt/CMR_DSMC_AutoSarNMNodeId ==
  in : Inport
  out : Outport
  wires:
  in/1 -> out/1

== system test_mdl_NI/CAN_Signal/DSMC/CMR_DSMC_AutoSar_NetwrkMgt/CMR_DSMC_AutoSarNMReserve2 ==
  in : Inport
  out : Outport
  wires:
  in/1 -> out/1

== system test_mdl_NI/CAN_Signal/DSMC/CMR_DSMC_AutoSar_NetwrkMgt/CMR_DSMC_AutoSarNMReserve3 ==
  in : Inport
  out : Outport
  wires:
  in/1 -> out/1

== system test_mdl_NI/CAN_Signal/DSMC/CMR_DSMC_AutoSar_NetwrkMgt/CMR_DSMC_AutoSarNMReserve4 ==
  in : Inport
  out : Outport
  wires:
  in/1 -> out/1

== system test_mdl_NI/CAN_Signal/DSMC/CMR_DSMC_AutoSar_NetwrkMgt/CMR_DSMC_AutoSarNMReserved ==
  in : Inport
  out : Outport
  wires:
  in/1 -> out/1

== system test_mdl_NI/CAN_Signal/DSMC/CMR_DSMC_AutoSar_NetwrkMgt/CMR_DSMC_GWNMProxY ==
  in : Inport
  out : Outport
  wires:
  in/1 -> out/1

== system test_mdl_NI/CAN_Signal/DSMC/CMR_DSMC_AutoSar_NetwrkMgt/CMR_DSMC_GWOnBoardTester ==
  in : Inport
  out : Outport
  wires:
  in/1 -> out/1

== system test_mdl_NI/CAN_Signal/DSMC/DrvStatMonData/DrvAlertSt_D_Stat ==
  in : Inport
  out : Outport
  wires:
  in/1 -> out/1

== system test_mdl_NI/CAN_Signal/DSMC/DrvStatMonData/DrvAttentZone_D_Stat ==
  in : Inport
  out : Outport
  wires:
  in/1 -> out/1

== system test_mdl_NI/CAN_Signal/DSMC/DrvStatMonData/DrvCamDrvIR_D_Stat ==
  in : Inport
  out : Outport
  wires:
  in/1 -> out/1

== system test_mdl_NI/CAN_Signal/DSMC/DrvStatMonData/DrvCamPassIR_D_Stat ==
  in : Inport
  out : Outport
  wires:
  in/1 -> out/1

== system test_mdl_NI/CAN_Signal/DSMC/DrvStatMonData/DrvCamera_D_Stat ==
  in : Inport
  out : Outport
  wires:
  in/1 -> out/1

== system test_mdl_NI/CAN_Signal/DSMC/DrvStatMonData/DrvEngLvlConfid_D_Stat ==
  in : Inport
  out : Outport
  wires:
  in/1 -> out/1

== system test_mdl_NI/CAN_Signal/DSMC/DrvStatMonData/DrvEngageLevel_D_Stat ==
  in : Inport
  out : Outport
  wires:
  in/1 -> out/1

== system test_mdl_NI/CAN_Signal/DSMC/DrvStatMonData/DrvEngageLevel_No_Cnt ==
  in : Inport
  out : Outport
  wires:
  in/1 -> out/1

== system test_mdl_NI/CAN_Signal/DSMC/DrvStatMonData/DrvEngageLevel_No_Cs ==
  in : Inport
  out : Outport
  wires:
  in/1 -> out/1

== system test_mdl_NI/CAN_Signal/DSMC/DrvStatMonData/DrvImpLvlConfid_D_Stat ==
  in : Inport
  out : Outport
  wires:
  in/1 -> out/1

== system test_mdl_NI/CAN_Signal/DSMC/DrvStatMonData/DrvImpairLvl_D_Stat ==
  in : Inport
  out : Outport
  wires:
  in/1 -> out/1

== system test_mdl_NI/CAN_Signal/DSMC/TesterPhysicalResCMR_DSMC/TesterPhysicalResCMR_DSMC ==
  in : Inport
  out : Outport
  wires:
  in/1 -> out/1

== system test_mdl_NI/CAN_Signal/ECM_DIESEL PCM PCM_HEV/EngBrakeData_0x165/AccEngStat_D_Actl ==
  in : Inport
  out : Outport
  wires:
  in/1 -> out/1

== system test_mdl_NI/CAN_Signal/ECM_DIESEL PCM PCM_HEV/EngBrakeData_0x165/AccStopMde_D_Rq ==
  in : Inport
  out : Outport
  wires:
  in/1 -> out/1

== system test_mdl_NI/CAN_Signal/ECM_DIESEL PCM PCM_HEV/EngBrakeData_0x165/BPedDrvAppl_D_QF ==
  in : Inport
  out : Outport
  wires:
  in/1 -> out/1

== system test_mdl_NI/CAN_Signal/ECM_DIESEL PCM PCM_HEV/EngBrakeData_0x165/BpedDrvAppl_D_Actl ==
  in : Inport
  out : Outport
  wires:
  in/1 -> out/1

== system test_mdl_NI/CAN_Signal/ECM_DIESEL PCM PCM_HEV/EngBrakeData_0x165/CcMde_D_Actl ==
  in : Inport
  out : Outport
  wires:
  in/1 -> out/1

== system test_mdl_NI/CAN_Signal/ECM_DIESEL PCM PCM_HEV/EngBrakeData_0x165/CcOvrrdActv_B_Actl ==
  in : Inport
  out : Outport
  wires:
  in/1 -> out/1

== system test_mdl_NI/CAN_Signal/ECM_DIESEL PCM PCM_HEV/EngBrakeData_0x165/CcStat_D_Actl ==
  in : Inport
  out : Outport
  wires:
  in/1 -> out/1

== system test_mdl_NI/CAN_Signal/ECM_DIESEL PCM PCM_HEV/EngBrakeData_0x165/CmbbDeny_B_ActlPrpl ==
  in : Inport
  out : Outport
  wires:
  in/1 -> out/1

== system test_mdl_NI/CAN_Signal/ECM_DIESEL PCM PCM_HEV/EngBrakeData_0x165/CmbbEngTqMn_B_Actl ==
  in : Inport
  out : Outport
  wires:
  in/1 -> out/1

== system test_mdl_NI/CAN_Signal/ECM_DIESEL PCM PCM_HEV/EngBrakeData_0x165/EngAout_N_MnAllw ==
  in : Inport
  out : Outport
  wires:
  in/1 -> out/1

== system test_mdl_NI/CAN_Signal/ECM_DIESEL PCM PCM_HEV/EngBrakeData_0x165/PrplTqMnSat_B_Actl ==
  in : Inport
  out : Outport
  wires:
  in/1 -> out/1

== system test_mdl_NI/CAN_Signal/ECM_DIESEL PCM PCM_HEV/EngBrakeData_0x165/Veh_V_DsplyCcSet ==
  in : Inport
  out : Outport
  wires:
  in/1 -> out/1

== system test_mdl_NI/CAN_Signal/ECM_DIESEL PCM PCM_HEV/EngVehicleSpThrottle2_0x202/GearRvrse_D_Actl ==
  in : Inport
  out : Outport
  wires:
  in/1 -> out/1

== system test_mdl_NI/CAN_Signal/ECM_DIESEL PCM PCM_HEV/EngVehicleSpThrottle2_0x202/StrtrMtrCtlMsgTxt_D2_Rq ==
  in : Inport
  out : Outport
  wires:
  in/1 -> out/1

== system test_mdl_NI/CAN_Signal/ECM_DIESEL PCM PCM_HEV/EngVehicleSpThrottle2_0x202/StrtrMtrCtlMsgTxt_D_Rq ==
  in : Inport
  out : Outport
  wires:
  in/1 -> out/1

== system test_mdl_NI/CAN_Signal/ECM_DIESEL PCM PCM_HEV/EngVehicleSpThrottle2_0x202/StrtrMtrDlyStrt_B_Stat ==
  in : Inport
  out : Outport
  wires:
  in/1 -> out/1

== system test_mdl_NI/CAN_Signal/ECM_DIESEL PCM PCM_HEV/EngVehicleSpThrottle2_0x202/VehVActlEng_D_Qf ==
  in : Inport
  out : Outport
  wires:
  in/1 -> out/1

== system test_mdl_NI/CAN_Signal/ECM_DIESEL PCM PCM_HEV/EngVehicleSpThrottle2_0x202/VehVActlEng_No_Cnt ==
  in : Inport
  out : Outport
  wires:
  in/1 -> out/1

== system test_mdl_NI/CAN_Signal/ECM_DIESEL PCM PCM_HEV/EngVehicleSpThrottle2_0x202/VehVActlEng_No_Cs ==
  in : Inport
  out : Outport
  wires:
  in/1 -> out/1

== system test_mdl_NI/CAN_Signal/ECM_DIESEL PCM PCM_HEV/EngVehicleSpThrottle2_0x202/VehVTrlrAid_B_Avail ==
  in : Inport
  out : Outport
  wires:
  in/1 -> out/1

== system test_mdl_NI/CAN_Signal/ECM_DIESEL PCM PCM_HEV/EngVehicleSpThrottle2_0x202/Veh_V_ActlEng ==
  in : Inport
  out : Outport
  wires:
  in/1 -> out/1

== system test_mdl_NI/CAN_Signal/ECM_DIESEL PCM PCM_HEV/EngVehicleSpThrottle2_0x202/Veh_V_RqCcSet ==
  in : Inport
  out : Outport
  wires:
  in/1 -> out/1

== system test_mdl_NI/CAN_Signal/ECM_DIESEL PCM PCM_HEV/EngVehicleSpThrottle_0x204/ApedPosPcActl_D_Qf ==
  in : Inport
  out : Outport
  wires:
  in/1 -> out/1

== system test_mdl_NI/CAN_Signal/ECM_DIESEL PCM PCM_HEV/EngVehicleSpThrottle_0x204/ApedPosPcActl_No_Cnt ==
  in : Inport
  out : Outport
  wires:
  in/1 -> out/1

== system test_mdl_NI/CAN_Signal/ECM_DIESEL PCM PCM_HEV/EngVehicleSpThrottle_0x204/ApedPosPcActl_No_Cs ==
  in : Inport
  out : Outport
  wires:
  in/1 -> out/1

== system test_mdl_NI/CAN_Signal/ECM_DIESEL PCM PCM_HEV/EngVehicleSpThrottle_0x204/ApedPos_PcRate_ActlArb ==
  in : Inport
  out : Outport
  wires:
  in/1 -> out/1

== system test_mdl_NI/CAN_Signal/ECM_DIESEL PCM PCM_HEV/EngVehicleSpThrottle_0x204/ApedPos_Pc_ActlArb ==
  in : Inport
  out : Outport
  wires:
  in/1 -> out/1

== system test_mdl_NI/CAN_Signal/ECM_DIESEL PCM PCM_HEV/EngVehicleSpThrottle_0x204/EngAout3_N_Actl ==
  in : Inport
  out : Outport
  wires:
  in/1 -> out/1

== system test_mdl_NI/CAN_Signal/ECM_DIESEL PCM PCM_HEV/EngVehicleSpThrottle_0x204/EngAoutNActl_D_QF ==
  in : Inport
  out : Outport
  wires:
  in/1 -> out/1

== system test_mdl_NI/CAN_Signal/ECM_DIESEL PCM PCM_HEV/EngVehicleSpThrottle_0x204/EngAout_N_Actl ==
  in : Inport
  out : Outport
  wires:
  in/1 -> out/1

== system test_mdl_NI/CAN_Signal/ECM_DIESEL PCM PCM_HEV/EngineClimateData_0x178/AirAmbTe_D_Qf ==
  in : Inport
  out : Outport
  wires:
  in/1 -> out/1

== system test_mdl_NI/CAN_Signal/ECM_DIESEL PCM PCM_HEV/EngineClimateData_0x178/AirAmb_P_Actl ==
  in : Inport
  out : Outport
  wires:
  in/1 -> out/1

== system test_mdl_NI/CAN_Signal/ECM_DIESEL PCM PCM_HEV/EngineClimateData_0x178/AirAmb_Te_Actl ==
  in : Inport
  out : Outport
  wires:
  in/1 -> out/1

== system test_mdl_NI/CAN_Signal/ECM_DIESEL PCM PCM_HEV/EngineClimateData_0x178/AirAmb_Te_ActlFilt ==
  in : Inport
  out : Outport
  wires:
  in/1 -> out/1

== system test_mdl_NI/CAN_Signal/ECM_DIESEL PCM PCM_HEV/EngineClimateData_0x178/AslChime_B_Rq ==
  in : Inport
  out : Outport
  wires:
  in/1 -> out/1

== system test_mdl_NI/CAN_Signal/ECM_DIESEL PCM PCM_HEV/EngineClimateData_0x178/AslIconDsply_D_Rq ==
  in : Inport
  out : Outport
  wires:
  in/1 -> out/1

== system test_mdl_NI/CAN_Signal/ECM_DIESEL PCM PCM_HEV/EngineClimateData_0x178/DynoMde_B_Cmd ==
  in : Inport
  out : Outport
  wires:
  in/1 -> out/1

== system test_mdl_NI/CAN_Signal/ECM_DIESEL PCM PCM_HEV/EngineClimateData_0x178/EcssLamp_D_RqDsply ==
  in : Inport
  out : Outport
  wires:
  in/1 -> out/1

== system test_mdl_NI/CAN_Signal/ECM_DIESEL PCM PCM_HEV/EngineClimateData_0x178/EngAout_Aa_Actl ==
  in : Inport
  out : Outport
  wires:
  in/1 -> out/1

== system test_mdl_NI/CAN_Signal/ECM_DIESEL PCM PCM_HEV/EngineClimateData_0x178/GasPrtc_D_RqDsply ==
  in : Inport
  out : Outport
  wires:
  in/1 -> out/1

== system test_mdl_NI/CAN_Signal/ECM_DIESEL PCM PCM_HEV/EngineClimateData_0x178/HvacHtrCore2_Te_Actl ==
  in : Inport
  out : Outport
  wires:
  in/1 -> out/1

== system test_mdl_NI/CAN_Signal/ECM_DIESEL PCM PCM_HEV/EngineData_6_0x156/EngClntTe_D_Qf ==
  in : Inport
  out : Outport
  wires:
  in/1 -> out/1

== system test_mdl_NI/CAN_Signal/ECM_DIESEL PCM PCM_HEV/EngineData_6_0x156/EngClnt_Te_Actl ==
  in : Inport
  out : Outport
  wires:
  in/1 -> out/1

== system test_mdl_NI/CAN_Signal/ECM_DIESEL PCM PCM_HEV/EngineData_6_0x156/EngGoutLss_Tq_Est ==
  in : Inport
  out : Outport
  wires:
  in/1 -> out/1

== system test_mdl_NI/CAN_Signal/ECM_DIESEL PCM PCM_HEV/EngineData_6_0x156/EngOil_Te_Actl ==
  in : Inport
  out : Outport
  wires:
  in/1 -> out/1

== system test_mdl_NI/CAN_Signal/ECM_DIESEL PCM PCM_HEV/EngineData_6_0x156/EngOvrhtMitgActv_D_Ind ==
  in : Inport
  out : Outport
  wires:
  in/1 -> out/1

== system test_mdl_NI/CAN_Signal/ECM_DIESEL PCM PCM_HEV/EngineData_7_0x179/AirCondClutch_B_Stats ==
  in : Inport
  out : Outport
  wires:
  in/1 -> out/1

== system test_mdl_NI/CAN_Signal/ECM_DIESEL PCM PCM_HEV/EngineData_7_0x179/AirCondRec_B_Rq ==
  in : Inport
  out : Outport
  wires:
  in/1 -> out/1

== system test_mdl_NI/CAN_Signal/ECM_DIESEL PCM PCM_HEV/EngineData_7_0x179/EngOilLife_Pc_Actl ==
  in : Inport
  out : Outport
  wires:
  in/1 -> out/1

== system test_mdl_NI/CAN_Signal/ECM_DIESEL PCM PCM_HEV/EngineData_7_0x179/EngSrvcRqd_B_Rq ==
  in : Inport
  out : Outport
  wires:
  in/1 -> out/1

== system test_mdl_NI/CAN_Signal/ECM_DIESEL PCM PCM_HEV/EngineData_7_0x179/FuelFillInlet_B_Dsply ==
  in : Inport
  out : Outport
  wires:
  in/1 -> out/1

== system test_mdl_NI/CAN_Signal/ECM_DIESEL PCM PCM_HEV/EngineData_7_0x179/FuelFilterLamp_B_Dsply ==
  in : Inport
  out : Outport
  wires:
  in/1 -> out/1
